simulink model "tdhdkHTbandau"  (R2016a)
settings: Solver=VariableStepAuto  StartTime=0.0  StopTime=10  RelTol=1e-3
undefined symbols (not defined in the file): bequiv, Jequiv, Kb, Kt, La, n, r, Ra
settings Model: Creator=Tuan  LastModifiedBy=Tuan

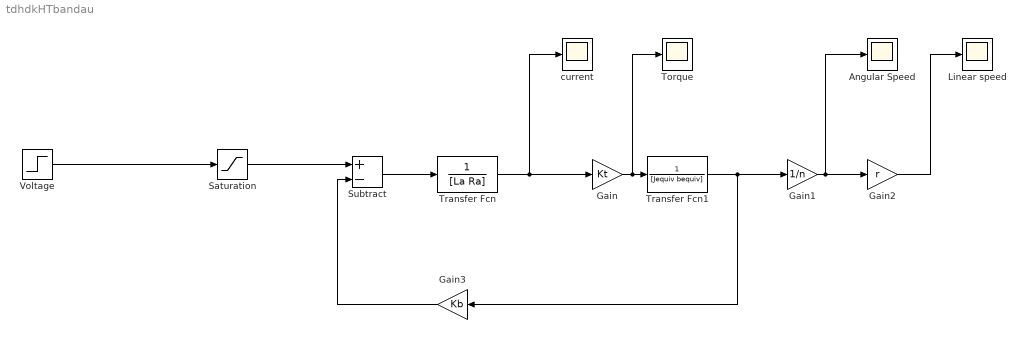
== system tdhdkHTbandau ==
  Angular Speed : Scope
  Gain : Gain  Gain=Kt
  Gain1 : Gain  Gain=1/n
  Gain2 : Gain  Gain=r
  Gain3 : Gain  Gain=Kb
  Linear speed : Scope
  Saturation : Saturate  UpperLimit=20  LowerLimit=-20
  Subtract : Sum  Inputs=+-
  Torque : Scope
  Transfer Fcn : TransferFcn  Denominator=[La Ra]
  Transfer Fcn1 : TransferFcn  Denominator=[Jequiv bequiv]
  Voltage : Step  Time=0  After=12  SampleTime=0
  current : Scope
  wires:
  Saturation/1 -> Subtract/1
  Subtract/1 -> Transfer Fcn/1
  Transfer Fcn/1 -> current/1, Gain/1
  Transfer Fcn1/1 -> Gain3/1, Gain1/1
  Gain1/1 -> Gain2/1, Angular Speed/1
  Gain2/1 -> Linear speed/1
  Gain3/1 -> Subtract/2
  Gain/1 -> Torque/1, Transfer Fcn1/1
  Voltage/1 -> Saturation/1
